simulink model "pddis"  (Simulink 3.00)
settings: Solver=ode5  SolverMode=SingleTasking  StartTime=0.0  StopTime=2.335  FixedStep=0.001  MaxStep=0.001  RelTol=1e-3  AbsTol=1e-3
values from neighbouring files (symbols this model uses):
  b = 5E-5    (= 5e-05)    [Constants.m]
  J = 1    [Constants.m]
  Ka = 20    [Constants.m]
  Km = 1.36    [Constants.m]
undefined symbols (not defined in the file or in its folder): a0, a1
settings Model: SaveTime=off  SaveOutput=off

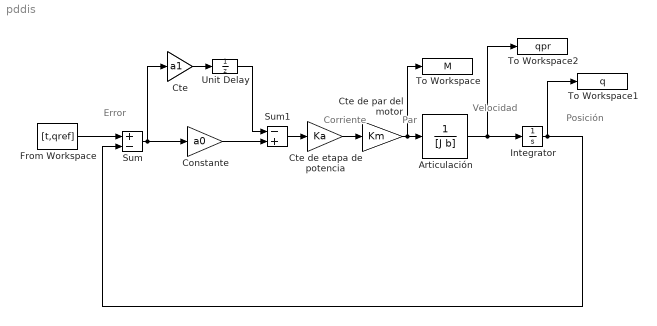
== system pddis ==
  note: Corriente
  note: Error
  note: Par
  note: Velocidad
  note: Posición
  Articulación : TransferFcn  Numerator=[1]  Denominator=[J b]
  Constante : Gain  Gain=a0  SaturateOnIntegerOverflow=on
  "Cte " : Gain  Gain=a1  SaturateOnIntegerOverflow=on
  Cte de etapa de potencia : Gain  Gain=Ka  SaturateOnIntegerOverflow=on
  Cte de par del motor : Gain  Gain=Km  SaturateOnIntegerOverflow=on
  From Workspace : FromWorkspace  VariableName=[t,qref]  SampleTime=0.001  HoldFinalValue=off
  Integrator : Integrator  ExternalReset=none  InitialConditionSource=internal  InitialCondition=0  LimitOutput=off  UpperSaturationLimit=inf  LowerSaturationLimit=-inf  ShowSaturationPort=off  ShowStatePort=off  AbsoluteTolerance=auto
  Sum : Sum  Inputs=+-  SaturateOnIntegerOverflow=on
  Sum1 : Sum  Inputs=-+  SaturateOnIntegerOverflow=on
  To Workspace : ToWorkspace  VariableName=M  SampleTime=0  SaveFormat=Matrix
      settings: Buffer=2335
  To Workspace1 : ToWorkspace  VariableName=q  SampleTime=0  SaveFormat=Matrix
      settings: Buffer=2335
  To Workspace2 : ToWorkspace  VariableName=qpr  SampleTime=0  SaveFormat=Matrix
      settings: Buffer=2335
  Unit Delay : UnitDelay  X0=0  SampleTime=0.001
  wires:
  Cte de etapa de potencia/1 -> Cte de par del motor/1
  From Workspace/1 -> Sum/1
  Cte de par del motor/1 -> Articulación/1, To Workspace/1
  Sum1/1 -> Cte de etapa de potencia/1
  Integrator/1 -> Sum/2, To Workspace1/1
  Articulación/1 -> Integrator/1, To Workspace2/1
  Constante/1 -> Sum1/2
  "Cte "/1 -> Unit Delay/1
  Sum/1 -> Constante/1, "Cte "/1
  Unit Delay/1 -> Sum1/1
